simulink subsystem "WP07_PW"  (R2021b)
settings: Solver=VariableStepAuto  StartTime=0.0  StopTime=10.0  RelTol=1e-3
values from neighbouring files (symbols this model uses):
  Ctx_dcr_eol_dcr = [0.002858 0.002047 0.001273 0.000905] * 1.1    [Cal_WP07_Power.m]
  Ctx_dcr_eol_temp = [0 10 25 45]    [Cal_WP07_Power.m]
  Ctx_pow_chg_drt_coef = [0     0    0    1 1  0]    [Cal_WP07_Power.m]
  Ctx_pow_chg_drt_temp = [-22 -21.9  2.9  3 51 52]    [Cal_WP07_Power.m]
  Ctx_pow_dch_drt_coef = [0     0    0    1 1  0]    [Cal_WP07_Power.m]
  Ctx_pow_dch_drt_temp = [-22 -21.9  -0.1  0 51 52]    [Cal_WP07_Power.m]
  Ctx_pow_dch_soc_neg_pow_lim = [128 132 136 143 156]    [Cal_WP07_Power.m]
  Ctx_pow_dch_soc_neg_pow_now = [0.1 0.2 0.33 0.5 1]*183    [Cal_WP07_Power.m]
  Cxx_1cp_str = 183    [Cal_WP07_Power.m]
  Cxx_cell_t_fbdn_dch = -22    [Cal_WP07_Power.m]
  Cxx_cell_v_cut_off_chg = 4.1    [Cal_WP07_Power.m]
  Cxx_cell_v_cut_off_dch = 3.025    [Cal_WP07_Power.m]
  Cxx_cell_v_cut_off_dch_lowt = 3.2    [Cal_WP07_Power.m]
  Cxx_cell_v_fbdn_chg = 4.11    [Cal_WP07_Power.m]
  Cxx_cell_v_fbdn_dch = 3.015    [Cal_WP07_Power.m]
  Cxx_dcpm_r = 0.0464    [Cal_WP07_Power.m]
  Cxx_i_thrd_chg_act = 1    [Cal_WP07_Power.m]
  Cxx_i_thrd_dch_act = -1    [Cal_WP07_Power.m]
  Cxx_low_dch_hyst_off = 0    [Cal_WP07_Power.m]
  Cxx_low_dch_hyst_on = 3    [Cal_WP07_Power.m]
  Cxx_low_dch_pow = 5.5    [Cal_WP07_Power.m]
  Cxx_pow_dir_cf_time = 0.1    [Cal_WP07_Power.m]
  Cxx_pow_dir_chg = 2    [Cal_WP07_Power.m]
  Cxx_pow_dir_dch = 3    [Cal_WP07_Power.m]
  Cxx_pow_dir_init = 0    [Cal_WP07_Power.m]
  Cxx_pow_dir_stb = 1    [Cal_WP07_Power.m]
  Cxx_sch_pw = 0.1    [Cal_WP07_Power.m]
  Cxx_str_i_abs_max = 168    [Cal_WP07_Power.m]
undefined symbols (not defined in the file or in its folder): Cxx_cell_per_str, Nxx_m_1, Nxx_w_2_kw
libraries: Lib_MBD_Ext x4, simulink_extras x2
settings Model: Creator=DoHieuTrinh  LastModifiedBy=DoHieuTrinh

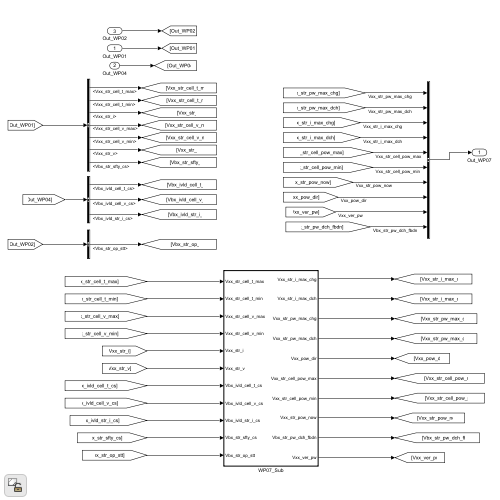
[thumbnail: Simulink's stored preview of the top-level diagram]
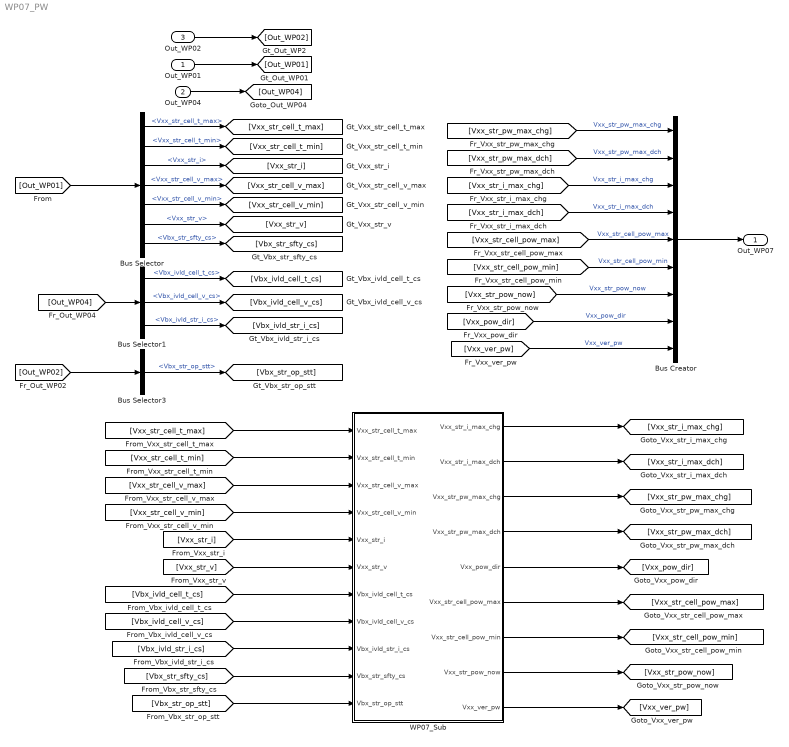
== system WP07_PW ==
  Out_WP01 : Inport
  Out_WP04 : Inport  Port=2
  Out_WP02 : Inport  Port=3
  Bus Creator : BusCreator  Inputs=9
  Bus Selector : BusSelector  OutputSignals=Vxx_str_cell_t_max,Vxx_str_cell_t_min,Vxx_str_i,Vxx_str_cell_v_max,Vxx_str_cell_v_min,Vxx_str_v,Vbx_str_sfty_cs
  Bus Selector1 : BusSelector  OutputSignals=Vbx_ivld_cell_t_cs,Vbx_ivld_cell_v_cs,Vbx_ivld_str_i_cs
  Bus Selector3 : BusSelector  OutputSignals=Vbx_str_op_stt
  WP07_Sub : Subsystem  TreatAsAtomicUnit=on  SystemSampleTime=0.1
  Out_WP07 : Outport
  wires:
  Bus Creator/1 -> Out_WP07/1
  [Vxx_str_pw_max_dch] -> Bus Creator/2  "Vxx_str_pw_max_dch"
  [Vxx_str_pw_max_chg] -> Bus Creator/1  "Vxx_str_pw_max_chg"
  [Out_WP01] -> Bus Selector/1
  Out_WP01/1 -> [Out_WP01]
  [Vxx_str_i_max_chg] -> Bus Creator/3  "Vxx_str_i_max_chg"
  [Vxx_str_i_max_dch] -> Bus Creator/4  "Vxx_str_i_max_dch"
  [Vxx_pow_dir] -> Bus Creator/8  "Vxx_pow_dir"
  WP07_Sub/1(Vxx_str_i_max_chg) -> [Vxx_str_i_max_chg]
  WP07_Sub/2(Vxx_str_i_max_dch) -> [Vxx_str_i_max_dch]
  WP07_Sub/3(Vxx_str_pw_max_chg) -> [Vxx_str_pw_max_chg]
  WP07_Sub/4(Vxx_str_pw_max_dch) -> [Vxx_str_pw_max_dch]
  WP07_Sub/5(Vxx_pow_dir) -> [Vxx_pow_dir]
  WP07_Sub/6(Vxx_str_cell_pow_max) -> [Vxx_str_cell_pow_max]
  WP07_Sub/7(Vxx_str_cell_pow_min) -> [Vxx_str_cell_pow_min]
  WP07_Sub/8(Vxx_str_pow_now) -> [Vxx_str_pow_now]
  [Vxx_str_cell_pow_max] -> Bus Creator/5  "Vxx_str_cell_pow_max"
  [Vxx_str_cell_pow_min] -> Bus Creator/6  "Vxx_str_cell_pow_min"
  [Vxx_str_pow_now] -> Bus Creator/7  "Vxx_str_pow_now"
  WP07_Sub/9(Vxx_ver_pw) -> [Vxx_ver_pw]
  [Vxx_ver_pw] -> Bus Creator/9  "Vxx_ver_pw"
  Out_WP04/1 -> [Out_WP04]
  [Out_WP04] -> Bus Selector1/1
  [Vxx_str_cell_t_max] -> WP07_Sub/1(Vxx_str_cell_t_max)
  [Vxx_str_cell_t_min] -> WP07_Sub/2(Vxx_str_cell_t_min)
  [Vxx_str_cell_v_max] -> WP07_Sub/3(Vxx_str_cell_v_max)
  [Vxx_str_cell_v_min] -> WP07_Sub/4(Vxx_str_cell_v_min)
  [Vxx_str_i] -> WP07_Sub/5(Vxx_str_i)
  [Vxx_str_v] -> WP07_Sub/6(Vxx_str_v)
  [Vbx_ivld_cell_t_cs] -> WP07_Sub/7(Vbx_ivld_cell_t_cs)
  [Vbx_ivld_cell_v_cs] -> WP07_Sub/8(Vbx_ivld_cell_v_cs)
  [Vbx_ivld_str_i_cs] -> WP07_Sub/9(Vbx_ivld_str_i_cs)
  Bus Selector/1 -> [Vxx_str_cell_t_max]  "<Vxx_str_cell_t_max>"
  Bus Selector/2 -> [Vxx_str_cell_t_min]  "<Vxx_str_cell_t_min>"
  Bus Selector/3 -> [Vxx_str_i]  "<Vxx_str_i>"
  Bus Selector/4 -> [Vxx_str_cell_v_max]  "<Vxx_str_cell_v_max>"
  Bus Selector/5 -> [Vxx_str_cell_v_min]  "<Vxx_str_cell_v_min>"
  Bus Selector/6 -> [Vxx_str_v]  "<Vxx_str_v>"
  Bus Selector1/1 -> [Vbx_ivld_cell_t_cs]  "<Vbx_ivld_cell_t_cs>"
  Bus Selector1/2 -> [Vbx_ivld_cell_v_cs]  "<Vbx_ivld_cell_v_cs>"
  Bus Selector1/3 -> [Vbx_ivld_str_i_cs]  "<Vbx_ivld_str_i_cs>"
  Bus Selector/7 -> [Vbx_str_sfty_cs]  "<Vbx_str_sfty_cs>"
  [Vbx_str_sfty_cs] -> WP07_Sub/10(Vbx_str_sfty_cs)
  [Vbx_str_op_stt] -> WP07_Sub/11(Vbx_str_op_stt)
  Bus Selector3/1 -> [Vbx_str_op_stt]  "<Vbx_str_op_stt>"
  [Out_WP02] -> Bus Selector3/1
  Out_WP02/1 -> [Out_WP02]

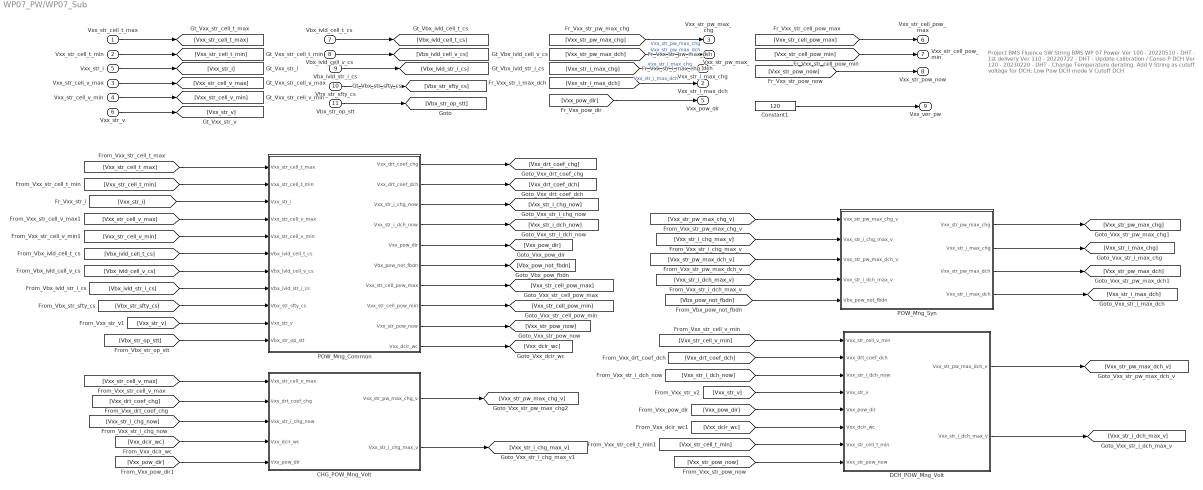
== system WP07_PW/WP07_Sub ==
  note: Project BMS Fluence
      | SW String BMS
      | WP 07 Power
      | Ver 100 - 20220510 - DHT - 1st delivery
      | Ver 110 - 20220722 - DHT - Update calibration / Conso P DCH
      | Ver 120 - 20230220 - DHT - Change Temperature derating.
      | Add V String as cutoff voltage for DCH; Low Pow DCH mode
      | V Cutoff DCH
  Vxx_str_cell_t_max : Inport
  Vxx_str_cell_t_min : Inport  Port=2
  Vxx_str_cell_v_max : Inport  Port=3
  Vxx_str_cell_v_min : Inport  Port=4
  Vxx_str_i : Inport  Port=5
  Vxx_str_v : Inport  Port=6
  Vbx_ivld_cell_t_cs : Inport  Port=7
  Vbx_ivld_cell_v_cs : Inport  Port=8
  Vbx_ivld_str_i_cs : Inport  Port=9
  Vbx_str_sfty_cs : Inport  Port=10
  Vbx_str_op_stt : Inport  Port=11
  CHG_POW_Mng_Volt : Subsystem
  Constant1 : Constant  Value=120  OutDataTypeStr=uint16
  DCH_POW_Mng_Volt : Subsystem
  POW_Mng_Common : Subsystem
  POW_Mng_Syn : Subsystem
  Vxx_str_i_max_chg : Outport
  Vxx_str_i_max_dch : Outport  Port=2
  Vxx_str_pw_max_chg : Outport  Port=3
  Vxx_str_pw_max_dch : Outport  Port=4
  Vxx_pow_dir : Outport  Port=5
  Vxx_str_cell_pow_max : Outport  Port=6
  Vxx_str_cell_pow_min : Outport  Port=7
  Vxx_str_pow_now : Outport  Port=8
  Vxx_ver_pw : Outport  Port=9
  wires:
  [Vxx_str_pow_now] -> DCH_POW_Mng_Volt/8(Vxx_str_pow_now)
  [Vxx_str_cell_t_min] -> DCH_POW_Mng_Volt/7(Vxx_str_cell_t_min)
  [Vxx_pow_dir] -> CHG_POW_Mng_Volt/5(Vxx_pow_dir)
  [Vxx_dcir_wc] -> DCH_POW_Mng_Volt/6(Vxx_dcir_wc)
  [Vxx_dcir_wc] -> CHG_POW_Mng_Volt/4(Vxx_dcir_wc)
  POW_Mng_Common/10(Vxx_dcir_wc) -> [Vxx_dcir_wc]
  [Vxx_pow_dir] -> DCH_POW_Mng_Volt/5(Vxx_pow_dir)
  [Vbx_str_op_stt] -> POW_Mng_Common/11(Vbx_str_op_stt)
  Vbx_str_op_stt/1 -> [Vbx_str_op_stt]
  [Vxx_str_v] -> POW_Mng_Common/10(Vxx_str_v)
  CHG_POW_Mng_Volt/2(Vxx_str_i_chg_max_v) -> [Vxx_str_i_chg_max_v]
  CHG_POW_Mng_Volt/1(Vxx_str_pw_max_chg_v) -> [Vxx_str_pw_max_chg_v]
  Vbx_str_sfty_cs/1 -> [Vbx_str_sfty_cs]
  [Vbx_str_sfty_cs] -> POW_Mng_Common/9(Vbx_str_sfty_cs)
  Vbx_ivld_str_i_cs/1 -> [Vbx_ivld_str_i_cs]
  Vbx_ivld_cell_v_cs/1 -> [Vbx_ivld_cell_v_cs]
  Vbx_ivld_cell_t_cs/1 -> [Vbx_ivld_cell_t_cs]
  [Vbx_ivld_str_i_cs] -> POW_Mng_Common/8(Vbx_ivld_str_i_cs)
  [Vbx_ivld_cell_v_cs] -> POW_Mng_Common/7(Vbx_ivld_cell_v_cs)
  [Vbx_ivld_cell_t_cs] -> POW_Mng_Common/6(Vbx_ivld_cell_t_cs)
  [Vxx_str_cell_v_min] -> POW_Mng_Common/5(Vxx_str_cell_v_min)
  [Vxx_str_cell_v_max] -> POW_Mng_Common/4(Vxx_str_cell_v_max)
  [Vxx_str_i] -> POW_Mng_Common/3(Vxx_str_i)
  [Vxx_str_cell_t_min] -> POW_Mng_Common/2(Vxx_str_cell_t_min)
  [Vxx_str_cell_t_max] -> POW_Mng_Common/1(Vxx_str_cell_t_max)
  Constant1/1 -> Vxx_ver_pw/1
  [Vxx_str_pow_now] -> Vxx_str_pow_now/1
  [Vxx_str_v] -> DCH_POW_Mng_Volt/4(Vxx_str_v)
  [Vxx_str_cell_pow_min] -> Vxx_str_cell_pow_min/1
  [Vxx_str_cell_pow_max] -> Vxx_str_cell_pow_max/1
  POW_Mng_Common/9(Vxx_str_pow_now) -> [Vxx_str_pow_now]
  POW_Mng_Common/8(Vxx_str_cell_pow_min) -> [Vxx_str_cell_pow_min]
  POW_Mng_Common/7(Vxx_str_cell_pow_max) -> [Vxx_str_cell_pow_max]
  [Vbx_pow_not_fbdn] -> POW_Mng_Syn/5(Vbx_pow_not_fbdn)
  POW_Mng_Common/6(Vbx_pow_not_fbdn) -> [Vbx_pow_not_fbdn]
  Vxx_str_v/1 -> [Vxx_str_v]
  [Vxx_pow_dir] -> Vxx_pow_dir/1
  POW_Mng_Common/5(Vxx_pow_dir) -> [Vxx_pow_dir]
  [Vxx_str_pw_max_dch] -> Vxx_str_pw_max_dch/1  "Vxx_str_pw_max_dch"
  [Vxx_str_pw_max_chg] -> Vxx_str_pw_max_chg/1  "Vxx_str_pw_max_chg"
  [Vxx_str_i_max_dch] -> Vxx_str_i_max_dch/1  "Vxx_str_i_max_dch"
  [Vxx_str_i_max_chg] -> Vxx_str_i_max_chg/1  "Vxx_str_i_max_chg"
  Vxx_str_i/1 -> [Vxx_str_i]
  Vxx_str_cell_v_min/1 -> [Vxx_str_cell_v_min]
  Vxx_str_cell_v_max/1 -> [Vxx_str_cell_v_max]
  Vxx_str_cell_t_min/1 -> [Vxx_str_cell_t_min]
  Vxx_str_cell_t_max/1 -> [Vxx_str_cell_t_max]
  [Vxx_drt_coef_dch] -> DCH_POW_Mng_Volt/2(Vxx_drt_coef_dch)
  POW_Mng_Syn/1(Vxx_str_pw_max_chg) -> [Vxx_str_pw_max_chg]
  POW_Mng_Syn/3(Vxx_str_pw_max_dch) -> [Vxx_str_pw_max_dch]
  POW_Mng_Common/3(Vxx_str_i_chg_now) -> [Vxx_str_i_chg_now]
  [Vxx_str_pw_max_dch_v] -> POW_Mng_Syn/3(Vxx_str_pw_max_dch_v)
  POW_Mng_Syn/2(Vxx_str_i_max_chg) -> [Vxx_str_i_max_chg]
  [Vxx_str_i_dch_max_v] -> POW_Mng_Syn/4(Vxx_str_i_dch_max_v)
  [Vxx_drt_coef_chg] -> CHG_POW_Mng_Volt/2(Vxx_drt_coef_chg)
  POW_Mng_Common/4(Vxx_str_i_dch_now) -> [Vxx_str_i_dch_now]
  [Vxx_str_pw_max_chg_v] -> POW_Mng_Syn/1(Vxx_str_pw_max_chg_v)
  [Vxx_str_i_chg_now] -> CHG_POW_Mng_Volt/3(Vxx_str_i_chg_now)
  [Vxx_str_i_dch_now] -> DCH_POW_Mng_Volt/3(Vxx_str_i_dch_now)
  POW_Mng_Syn/4(Vxx_str_i_max_dch) -> [Vxx_str_i_max_dch]
  [Vxx_str_i_chg_max_v] -> POW_Mng_Syn/2(Vxx_str_i_chg_max_v)
  POW_Mng_Common/1(Vxx_drt_coef_chg) -> [Vxx_drt_coef_chg]
  POW_Mng_Common/2(Vxx_drt_coef_dch) -> [Vxx_drt_coef_dch]
  DCH_POW_Mng_Volt/1(Vxx_str_pw_max_dch_v) -> [Vxx_str_pw_max_dch_v]
  DCH_POW_Mng_Volt/2(Vxx_str_i_dch_max_v) -> [Vxx_str_i_dch_max_v]
  [Vxx_str_cell_v_min] -> DCH_POW_Mng_Volt/1(Vxx_str_cell_v_min)
  [Vxx_str_cell_v_max] -> CHG_POW_Mng_Volt/1(Vxx_str_cell_v_max)

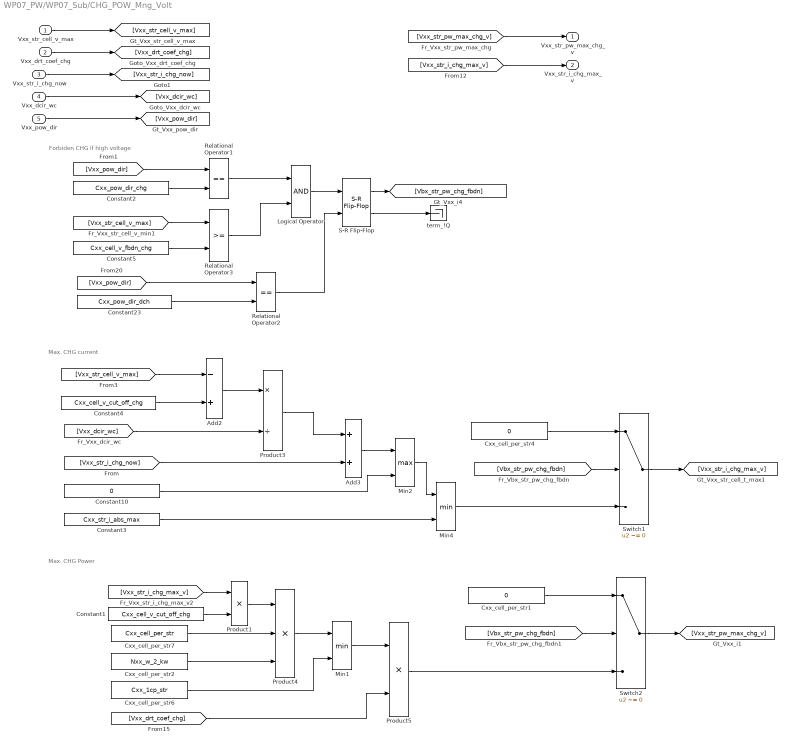
== system WP07_PW/WP07_Sub/CHG_POW_Mng_Volt ==
  note: Max. CHG current
  note: Max. CHG Power
  note: Forbiden CHG if high voltage
  Vxx_str_cell_v_max : Inport
  Vxx_drt_coef_chg : Inport  Port=2
  Vxx_str_i_chg_now : Inport  Port=3
  Vxx_dcir_wc : Inport  Port=4
  Vxx_pow_dir : Inport  Port=5
  Add2 : Sum  Inputs=-+
  Add3 : Sum
  Constant1 : Constant  Value=Cxx_cell_v_cut_off_chg  OutDataTypeStr=Inherit: Inherit via back propagation
  Constant10 : Constant  Value=0  OutDataTypeStr=Inherit: Inherit via back propagation
  Constant2 : Constant  Value=Cxx_pow_dir_chg  OutDataTypeStr=Inherit: Inherit via back propagation
  Constant23 : Constant  Value=Cxx_pow_dir_dch  OutDataTypeStr=Inherit: Inherit via back propagation
  Constant3 : Constant  Value=Cxx_str_i_abs_max  OutDataTypeStr=Inherit: Inherit via back propagation
  Constant4 : Constant  Value=Cxx_cell_v_cut_off_chg  OutDataTypeStr=Inherit: Inherit via back propagation
  Constant5 : Constant  Value=Cxx_cell_v_fbdn_chg  OutDataTypeStr=Inherit: Inherit via back propagation
  Cxx_cell_per_str1 : Constant  Value=0
  Cxx_cell_per_str2 : Constant  Value=Nxx_w_2_kw
  Cxx_cell_per_str4 : Constant  Value=0
  Cxx_cell_per_str6 : Constant  Value=Cxx_1cp_str
  Cxx_cell_per_str7 : Constant  Value=Cxx_cell_per_str
  Logical Operator : Logic  AllPortsSameDT=off  OutDataTypeStr=boolean
  Min1 : MinMax  Inputs=2
  Min2 : MinMax  Function=max  Inputs=2
  Min4 : MinMax  Inputs=2
  Product1 : Product
  Product3 : Product  Inputs=*/
  Product4 : Product  Inputs=3
  Product5 : Product
  Relational Operator1 : RelationalOperator  Operator===  OutDataTypeStr=boolean  RndMeth=Simplest
  Relational Operator2 : RelationalOperator  Operator===  OutDataTypeStr=boolean  RndMeth=Simplest
  Relational Operator3 : RelationalOperator  OutDataTypeStr=boolean  RndMeth=Simplest
  S-R Flip-Flop : simulink_extras/Flip Flops/S-R Flip-Flop  initial_condition=0
  Switch1 : Switch  Criteria=u2 ~= 0
  Switch2 : Switch  Criteria=u2 ~= 0
  term_!Q : Terminator
  Vxx_str_pw_max_chg_v : Outport
  Vxx_str_i_chg_max_v : Outport  Port=2
  wires:
  Relational Operator3/1 -> Logical Operator/2
  Product5/1 -> Switch2/3
  Switch2/1 -> [Vxx_str_pw_max_chg_v]
  Switch1/1 -> [Vxx_str_i_chg_max_v]
  [Vbx_str_pw_chg_fbdn] -> Switch2/2
  Cxx_cell_per_str1/1 -> Switch2/1
  Cxx_cell_per_str4/1 -> Switch1/1
  [Vbx_str_pw_chg_fbdn] -> Switch1/2
  Vxx_pow_dir/1 -> [Vxx_pow_dir]
  [Vxx_pow_dir] -> Relational Operator2/1
  [Vxx_str_cell_v_max] -> Relational Operator3/1
  Constant23/1 -> Relational Operator2/2
  Relational Operator2/1 -> S-R Flip-Flop/2
  Constant2/1 -> Relational Operator1/2
  S-R Flip-Flop/1 -> [Vbx_str_pw_chg_fbdn]
  S-R Flip-Flop/2 -> term_!Q/1
  [Vxx_pow_dir] -> Relational Operator1/1
  Logical Operator/1 -> S-R Flip-Flop/1
  Relational Operator1/1 -> Logical Operator/1
  Constant5/1 -> Relational Operator3/2
  Vxx_dcir_wc/1 -> [Vxx_dcir_wc]
  [Vxx_str_cell_v_max] -> Add2/1
  [Vxx_drt_coef_chg] -> Product5/2
  Min1/1 -> Product5/1
  Product4/1 -> Min1/1
  Cxx_cell_per_str2/1 -> Product4/3
  Cxx_cell_per_str7/1 -> Product4/2
  Product1/1 -> Product4/1
  Constant1/1 -> Product1/2
  [Vxx_str_i_chg_max_v] -> Product1/1
  Cxx_cell_per_str6/1 -> Min1/2
  Constant3/1 -> Min4/2
  Vxx_str_i_chg_now/1 -> [Vxx_str_i_chg_now]
  [Vxx_str_i_chg_max_v] -> Vxx_str_i_chg_max_v/1
  Vxx_drt_coef_chg/1 -> [Vxx_drt_coef_chg]
  Product3/1 -> Add3/1
  Vxx_str_cell_v_max/1 -> [Vxx_str_cell_v_max]
  Constant4/1 -> Add2/2
  [Vxx_dcir_wc] -> Product3/2
  Add2/1 -> Product3/1
  [Vxx_str_i_chg_now] -> Add3/2
  Add3/1 -> Min2/1
  Constant10/1 -> Min2/2
  [Vxx_str_pw_max_chg_v] -> Vxx_str_pw_max_chg_v/1
  Min4/1 -> Switch1/3
  Min2/1 -> Min4/1

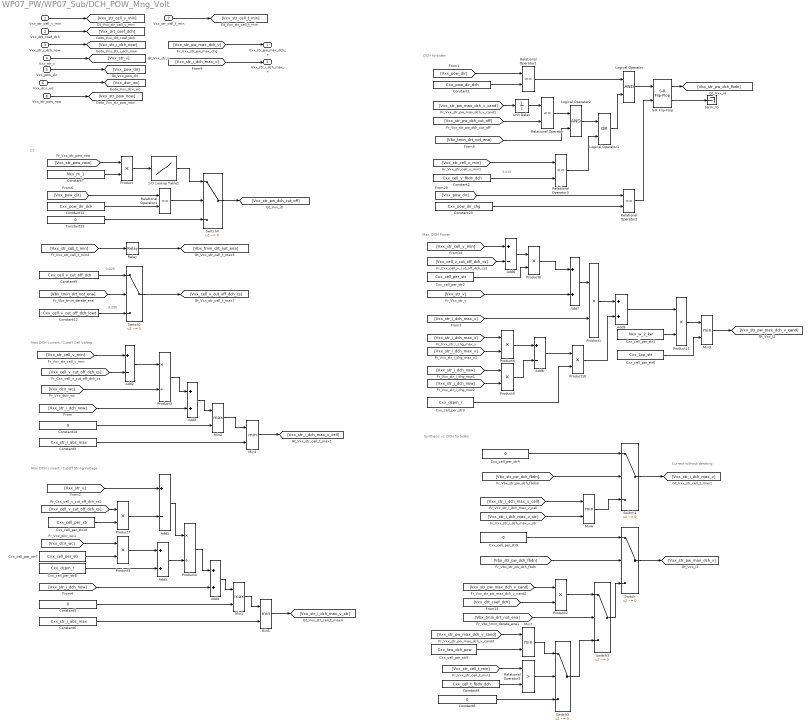
== system WP07_PW/WP07_Sub/DCH_POW_Mng_Volt ==
  note: Max DCH current / Cutoff String Voltage
  note: Max DCH current / Cutoff Cell Voltag
  note: Max. DCH Power
  note: DCH forbiden
  note: Synthesis vs. DCH forbiden
  note: CS
  note: Current without derating
  note: 3.015
  note: 3.025
  note: 3.200
  Vxx_str_cell_v_min : Inport
  Vxx_drt_coef_dch : Inport  Port=2
  Vxx_str_i_dch_now : Inport  Port=3
  Vxx_str_v : Inport  Port=4
  Vxx_pow_dir : Inport  Port=5
  Vxx_dcir_wc : Inport  Port=6
  Vxx_str_cell_t_min : Inport  Port=7
  Vxx_str_pow_now : Inport  Port=8
  1-D Lookup Table1 : Lookup_n-D  NumberOfTableDimensions=1  BreakpointsForDimension1=Ctx_pow_dch_soc_neg_pow_now  Table=Ctx_pow_dch_soc_neg_pow_lim  ExtrapMethod=Clip  UseLastTableValue=on  InternalRulePriority=Speed  RndMeth=Simplest  InputSameDT=on
  Add{1..2,6,8} (4 alike) : Sum  Inputs=+-
  Add{3..5,7,9} (5 alike) : Sum
  Constant1 : Constant  Value=Cxx_pow_dir_dch  OutDataTypeStr=Inherit: Inherit via back propagation
  Constant{5,8,10,13} (4 alike) : Constant  Value=0  OutDataTypeStr=Inherit: Inherit via back propagation
  Constant11 : Constant  Value=Cxx_pow_dir_dch  OutDataTypeStr=Inherit: Inherit via back propagation
  Constant12 : Constant  Value=Cxx_cell_v_cut_off_dch_lowt
  Constant2 : Constant  Value=Cxx_cell_v_fbdn_dch  OutDataTypeStr=Inherit: Inherit via back propagation
  Constant23 : Constant  Value=Cxx_pow_dir_chg  OutDataTypeStr=Inherit: Inherit via back propagation
  Constant3 : Constant  Value=Cxx_str_i_abs_max  OutDataTypeStr=Inherit: Inherit via back propagation
  Constant4 : Constant  Value=Cxx_cell_t_fbdn_dch  OutDataTypeStr=Inherit: Inherit via back propagation
  Constant6 : Constant  Value=Cxx_str_i_abs_max  OutDataTypeStr=Inherit: Inherit via back propagation
  Constant7 : Constant  Value=Nxx_m_1  OutDataTypeStr=Inherit: Inherit via back propagation
  Constant9 : Constant  Value=Cxx_cell_v_cut_off_dch
  Cxx_cell_per_str1 : Constant  Value=Nxx_w_2_kw
  Cxx_cell_per_str10 : Constant  Value=Cxx_cell_per_str
  Cxx_cell_per_str2 : Constant  Value=Cxx_cell_per_str
  Cxx_cell_per_str3 : Constant  Value=Cxx_dcpm_r
  Cxx_cell_per_str4 : Constant  Value=0
  Cxx_cell_per_str5 : Constant  Value=Cxx_low_dch_pow
  Cxx_cell_per_str6 : Constant  Value=Cxx_1cp_str
  Cxx_cell_per_str7 : Constant  Value=Cxx_cell_per_str
  Cxx_cell_per_str8 : Constant  Value=Cxx_dcpm_r
  Cxx_cell_per_str9 : Constant  Value=0
  Logical Operator : Logic  AllPortsSameDT=off  OutDataTypeStr=boolean
  Logical Operator1 : Logic  Operator=OR  AllPortsSameDT=off  OutDataTypeStr=boolean
  Logical Operator2 : Logic  AllPortsSameDT=off  OutDataTypeStr=boolean
  Min1 : MinMax  Function=max  Inputs=2
  Min2 : MinMax  Function=max  Inputs=2
  Min{3..7} (5 alike) : MinMax  Inputs=2
  Product{,1..2,5..11} (10 alike) : Product
  Product3 : Product  Inputs=*/
  Product4 : Product  Inputs=*/
  Relational Operator : RelationalOperator  Operator=<=  OutDataTypeStr=boolean  RndMeth=Simplest
  Relational Operator1 : RelationalOperator  Operator===  OutDataTypeStr=boolean  RndMeth=Simplest
  Relational Operator2 : RelationalOperator  Operator===  OutDataTypeStr=boolean  RndMeth=Simplest
  Relational Operator3 : RelationalOperator  Operator=<=  OutDataTypeStr=boolean  RndMeth=Simplest
  Relational Operator4 : RelationalOperator  Operator===  OutDataTypeStr=boolean  RndMeth=Simplest
  Relational Operator5 : RelationalOperator  Operator=>  OutDataTypeStr=boolean  RndMeth=Simplest
  Relay : Relay  OnSwitchValue=Cxx_low_dch_hyst_on  OffSwitchValue=Cxx_low_dch_hyst_off  OnOutputValue=true  OffOutputValue=false
  S-R Flip-Flop : simulink_extras/Flip Flops/S-R Flip-Flop  initial_condition=0
  Switch{,1..5} (6 alike) : Switch  Criteria=u2 ~= 0
  Unit Delay : UnitDelay  SampleTime=-1  HasFrameUpgradeWarning=on
  term_!Q : Terminator
  Vxx_str_pw_max_dch_v : Outport
  Vxx_str_i_dch_max_v : Outport  Port=2
  wires:
  Constant7/1 -> Product/2
  Product/1 -> 1-D Lookup Table1/1
  [Vxx_cell_v_cut_off_dch_cs] -> Add6/2
  Switch5/1 -> Switch3/3
  Constant8/1 -> Switch5/3
  Min7/1 -> Switch5/1
  Relational Operator5/1 -> Switch5/2
  [Vxx_str_cell_t_min] -> Relational Operator5/1
  Constant4/1 -> Relational Operator5/2
  [Vxx_str_pw_dch_cut_off] -> Relational Operator/2
  Switch4/1 -> [Vxx_str_pw_dch_cut_off]
  1-D Lookup Table1/1 -> Switch4/1
  [Vxx_str_pow_now] -> Product/1
  Constant13/1 -> Switch4/3
  Relational Operator4/1 -> Switch4/2
  Constant11/1 -> Relational Operator4/2
  [Vxx_pow_dir] -> Relational Operator4/1
  Vxx_str_pow_now/1 -> [Vxx_str_pow_now]
  Constant2/1 -> Relational Operator3/2
  [Vxx_cell_v_cut_off_dch_cs] -> Product7/1
  Cxx_cell_per_str10/1 -> Product7/2
  Logical Operator2/1 -> Logical Operator1/1
  [Vbx_tmin_drt_not_ena] -> Logical Operator2/2
  Relational Operator/1 -> Logical Operator2/1
  Switch3/1 -> Switch/3
  Cxx_cell_per_str5/1 -> Min7/2
  [Vxx_str_pw_max_dch_v_cand] -> Min7/1
  Product2/1 -> Switch3/1
  [Vxx_str_pw_max_dch_v_cand] -> Product2/1
  [Vbx_tmin_drt_not_ena] -> Switch3/2
  Min3/1 -> [Vxx_str_pw_max_dch_v_cand]
  [Vbx_tmin_drt_not_ena] -> Switch2/2
  Relay/1 -> [Vbx_tmin_drt_not_ena]
  [Vxx_cell_v_cut_off_dch_cs] -> Add2/2
  Vxx_str_cell_t_min/1 -> [Vxx_str_cell_t_min]
  Constant9/1 -> Switch2/1
  Switch2/1 -> [Vxx_cell_v_cut_off_dch_cs]
  Constant12/1 -> Switch2/3
  [Vxx_str_cell_t_min] -> Relay/1
  Min6/1 -> Switch1/3
  [Vxx_str_i_dch_max_v_cell] -> Min6/1
  [Vxx_str_i_dch_max_v_str] -> Min6/2
  Add5/1 -> Product4/2
  [Vxx_dcir_wc] -> Product5/1
  Product5/1 -> Add5/1
  Cxx_cell_per_str8/1 -> Add5/2
  Cxx_cell_per_str7/1 -> Product5/2
  Min1/1 -> Min5/1
  [Vxx_str_i_dch_now] -> Add4/2
  Constant5/1 -> Min1/2
  Constant6/1 -> Min5/2
  Min5/1 -> [Vxx_str_i_dch_max_v_str]
  Add4/1 -> Min1/1
  Product7/1 -> Add1/2
  Add1/1 -> Product4/1
  [Vxx_str_v] -> Add1/1
  Product4/1 -> Add4/1
  [Vxx_drt_coef_dch] -> Product2/2
  Unit Delay/1 -> Relational Operator/1
  [Vxx_str_pw_max_dch_v_cand] -> Unit Delay/1
  Switch1/1 -> [Vxx_str_i_dch_max_v]
  Cxx_cell_per_str4/1 -> Switch1/1
  [Vbx_str_pw_dch_fbdn] -> Switch1/2
  Logical Operator1/1 -> Logical Operator/2
  Relational Operator3/1 -> Logical Operator1/2
  [Vxx_str_cell_v_min] -> Relational Operator3/1
  Vxx_dcir_wc/1 -> [Vxx_dcir_wc]
  [Vbx_str_pw_dch_fbdn] -> Switch/2
  S-R Flip-Flop/1 -> [Vbx_str_pw_dch_fbdn]
  S-R Flip-Flop/2 -> term_!Q/1
  Logical Operator/1 -> S-R Flip-Flop/1
  Relational Operator1/1 -> Logical Operator/1
  [Vxx_pow_dir] -> Relational Operator1/1
  Constant1/1 -> Relational Operator1/2
  Vxx_pow_dir/1 -> [Vxx_pow_dir]
  Relational Operator2/1 -> S-R Flip-Flop/2
  Cxx_cell_per_str9/1 -> Switch/1
  Constant23/1 -> Relational Operator2/2
  [Vxx_pow_dir] -> Relational Operator2/1
  [Vxx_str_cell_v_min] -> Add2/1
  Switch/1 -> [Vxx_str_pw_max_dch_v]
  Product11/1 -> Min3/1
  Cxx_cell_per_str6/1 -> Min3/2
  Cxx_cell_per_str2/1 -> Product6/2
  Product6/1 -> Add7/1
  Add6/1 -> Product6/1
  Vxx_str_v/1 -> [Vxx_str_v]
  Cxx_cell_per_str3/1 -> Product10/2
  [Vxx_str_i_dch_now] -> Product9/1
  [Vxx_str_i_dch_max_v] -> Product1/2
  Product1/1 -> Add9/1
  [Vxx_str_i_dch_now] -> Product9/2
  Cxx_cell_per_str1/1 -> Product11/2
  Product8/1 -> Add8/1
  [Vxx_str_i_dch_max_v] -> Product8/1
  Add8/1 -> Product10/1
  [Vxx_str_v] -> Add7/2
  Product9/1 -> Add8/2
  [Vxx_str_i_dch_max_v] -> Product8/2
  Add7/1 -> Product1/1
  Add9/1 -> Product11/1
  Product10/1 -> Add9/2
  [Vxx_str_cell_v_min] -> Add6/1
  Constant3/1 -> Min4/2
  [Vxx_str_i_dch_max_v] -> Vxx_str_i_dch_max_v/1
  Vxx_str_i_dch_now/1 -> [Vxx_str_i_dch_now]
  Vxx_drt_coef_dch/1 -> [Vxx_drt_coef_dch]
  [Vxx_str_pw_max_dch_v] -> Vxx_str_pw_max_dch_v/1
  Constant10/1 -> Min2/2
  Add3/1 -> Min2/1
  [Vxx_str_i_dch_now] -> Add3/2
  Product3/1 -> Add3/1
  Add2/1 -> Product3/1
  [Vxx_dcir_wc] -> Product3/2
  Vxx_str_cell_v_min/1 -> [Vxx_str_cell_v_min]
  Min2/1 -> Min4/1
  Min4/1 -> [Vxx_str_i_dch_max_v_cell]

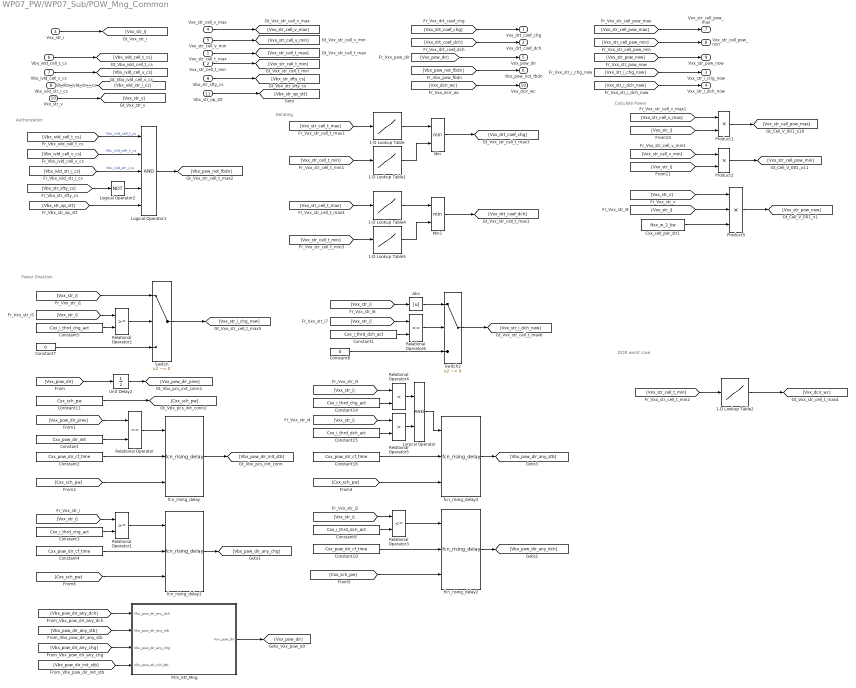
== system WP07_PW/WP07_Sub/POW_Mng_Common ==
  note: Calculate Power
  note: Derating
  note: Authorization
  note: Power Direction
  note: DCIR worst case
  Vxx_str_cell_t_max : Inport
  Vxx_str_cell_t_min : Inport  Port=2
  Vxx_str_i : Inport  Port=3
  Vxx_str_cell_v_max : Inport  Port=4
  Vxx_str_cell_v_min : Inport  Port=5
  Vbx_ivld_cell_t_cs : Inport  Port=6
  Vbx_ivld_cell_v_cs : Inport  Port=7
  Vbx_ivld_str_i_cs : Inport  Port=8
  Vbx_str_sfty_cs : Inport  Port=9
  Vxx_str_v : Inport  Port=10
  Vbx_str_op_stt : Inport  Port=11
  1-D Lookup Table : Lookup_n-D  NumberOfTableDimensions=1  BreakpointsForDimension1=Ctx_pow_chg_drt_temp  Table=Ctx_pow_chg_drt_coef  ExtrapMethod=Clip  UseLastTableValue=on  InternalRulePriority=Speed  RndMeth=Simplest  InputSameDT=on
  1-D Lookup Table1 : Lookup_n-D  NumberOfTableDimensions=1  BreakpointsForDimension1=Ctx_pow_chg_drt_temp  Table=Ctx_pow_chg_drt_coef  ExtrapMethod=Clip  UseLastTableValue=on  InternalRulePriority=Speed  RndMeth=Simplest  InputSameDT=on
  1-D Lookup Table2 : Lookup_n-D  NumberOfTableDimensions=1  BreakpointsForDimension1=Ctx_dcr_eol_temp  Table=Ctx_dcr_eol_dcr  ExtrapMethod=Clip  UseLastTableValue=on  InternalRulePriority=Speed  RndMeth=Simplest  InputSameDT=on
  1-D Lookup Table4 : Lookup_n-D  NumberOfTableDimensions=1  BreakpointsForDimension1=Ctx_pow_dch_drt_temp  Table=Ctx_pow_dch_drt_coef  ExtrapMethod=Clip  UseLastTableValue=on  InternalRulePriority=Speed  RndMeth=Simplest  InputSameDT=on
  1-D Lookup Table5 : Lookup_n-D  NumberOfTableDimensions=1  BreakpointsForDimension1=Ctx_pow_dch_drt_temp  Table=Ctx_pow_dch_drt_coef  ExtrapMethod=Clip  UseLastTableValue=on  InternalRulePriority=Speed  RndMeth=Simplest  InputSameDT=on
  Abs : Abs
  Constant : Constant  Value=Cxx_pow_dir_init
  Constant1 : Constant  Value=Cxx_i_thrd_dch_act
  Constant{2,4,10,16} (4 alike) : Constant  Value=Cxx_pow_dir_cf_time
  Constant11 : Constant  Value=Cxx_sch_pw
  Constant14 : Constant  Value=Cxx_i_thrd_chg_act
  Constant15 : Constant  Value=Cxx_i_thrd_dch_act
  Constant3 : Constant  Value=Cxx_i_thrd_chg_act
  Constant5 : Constant  Value=Cxx_i_thrd_chg_act
  Constant6 : Constant  Value=0
  Constant7 : Constant  Value=0
  Constant9 : Constant  Value=Cxx_i_thrd_dch_act
  Cxx_cell_per_str1 : Constant  Value=Nxx_w_2_kw
  Logical Operator : Logic  AllPortsSameDT=off  OutDataTypeStr=boolean
  Logical Operator1 : Logic  Inputs=5  AllPortsSameDT=off  OutDataTypeStr=boolean
  Logical Operator2 : Logic  Operator=NOT  AllPortsSameDT=off  OutDataTypeStr=boolean
  Min : MinMax  Inputs=2
  Min1 : MinMax  Inputs=2
  PCS_Stt_Mng : Stateflow chart  TreatAsAtomicUnit=on
  Product1 : Product
  Product2 : Product
  Product5 : Product  Inputs=3
  Relational Operator : RelationalOperator  Operator===  OutDataTypeStr=boolean  RndMeth=Simplest
  Relational Operator1 : RelationalOperator  OutDataTypeStr=boolean  RndMeth=Simplest
  Relational Operator2 : RelationalOperator  OutDataTypeStr=boolean  RndMeth=Simplest
  Relational Operator3 : RelationalOperator  Operator=<=  OutDataTypeStr=boolean  RndMeth=Simplest
  Relational Operator4 : RelationalOperator  Operator=<  OutDataTypeStr=boolean  RndMeth=Simplest
  Relational Operator5 : RelationalOperator  Operator=>  OutDataTypeStr=boolean  RndMeth=Simplest
  Relational Operator6 : RelationalOperator  Operator=<=  OutDataTypeStr=boolean  RndMeth=Simplest
  Switch : Switch  Criteria=u2 ~= 0
  Switch2 : Switch  Criteria=u2 ~= 0
  Unit Delay2 : UnitDelay  SampleTime=-1  HasFrameUpgradeWarning=on
  fcn_rising_delay{,1..3} (4 alike) : Lib_MBD_Ext/Timer/fcn_rising_delay  SystemSampleTime=-1  VariantActivationTime=update diagram  Latency=0  AutoFrameSizeCalculation=off
  Vxx_drt_coef_chg : Outport
  Vxx_drt_coef_dch : Outport  Port=2
  Vxx_str_i_chg_now : Outport  Port=3
  Vxx_str_i_dch_now : Outport  Port=4
  Vxx_pow_dir : Outport  Port=5
  Vbx_pow_not_fbdn : Outport  Port=6
  Vxx_str_cell_pow_max : Outport  Port=7
  Vxx_str_cell_pow_min : Outport  Port=8
  Vxx_str_pow_now : Outport  Port=9
  Vxx_dcir_wc : Outport  Port=10
  wires:
  Product5/1 -> [Vxx_str_pow_now]
  Cxx_cell_per_str1/1 -> Product5/3
  [Vxx_dcir_wc] -> Vxx_dcir_wc/1
  1-D Lookup Table2/1 -> [Vxx_dcir_wc]
  [Vxx_str_cell_t_min] -> 1-D Lookup Table2/1
  Constant1/1 -> Relational Operator6/2
  [Vxx_str_i] -> Relational Operator6/1
  Relational Operator2/1 -> Switch/2
  [Vxx_str_i] -> Relational Operator2/1
  Constant5/1 -> Relational Operator2/2
  [Vbx_str_op_stt] -> Logical Operator1/5
  Vbx_str_op_stt/1 -> [Vbx_str_op_stt]
  Constant11/1 -> [Cxx_sch_pw]
  Constant6/1 -> Switch2/3
  Abs/1 -> Switch2/1
  Vxx_str_v/1 -> [Vxx_str_v]
  [Vxx_str_v] -> Product5/1
  Logical Operator2/1 -> Logical Operator1/4
  [Vbx_str_sfty_cs] -> Logical Operator2/1
  Vbx_str_sfty_cs/1 -> [Vbx_str_sfty_cs]
  Vbx_ivld_str_i_cs/1 -> [Vbx_ivld_str_i_cs]
  Vbx_ivld_cell_v_cs/1 -> [Vbx_ivld_cell_v_cs]
  Vbx_ivld_cell_t_cs/1 -> [Vbx_ivld_cell_t_cs]
  [Vbx_ivld_str_i_cs] -> Logical Operator1/3  "Vbx_ivld_str_i_cs"
  [Vbx_ivld_cell_v_cs] -> Logical Operator1/2  "Vbx_ivld_cell_v_cs"
  [Vbx_ivld_cell_t_cs] -> Logical Operator1/1  "Vbx_ivld_cell_t_cs"
  [Vxx_str_i] -> Product5/2
  [Vxx_str_pow_now] -> Vxx_str_pow_now/1
  [Vxx_str_cell_pow_min] -> Vxx_str_cell_pow_min/1
  [Vxx_str_cell_pow_max] -> Vxx_str_cell_pow_max/1
  Vxx_str_cell_v_min/1 -> [Vxx_str_cell_v_min]
  Vxx_str_cell_v_max/1 -> [Vxx_str_cell_v_max]
  Product2/1 -> [Vxx_str_cell_pow_min]
  [Vxx_str_i] -> Product1/2
  [Vxx_str_cell_v_min] -> Product2/1
  [Vxx_str_i] -> Product2/2
  [Vxx_str_cell_v_max] -> Product1/1
  Product1/1 -> [Vxx_str_cell_pow_max]
  [Vbx_pow_not_fbdn] -> Vbx_pow_not_fbdn/1
  Logical Operator1/1 -> [Vbx_pow_not_fbdn]
  [Vxx_pow_dir] -> Vxx_pow_dir/1
  [Vxx_str_i_dch_now] -> Vxx_str_i_dch_now/1
  [Vxx_str_i_chg_now] -> Vxx_str_i_chg_now/1
  Relational Operator6/1 -> Switch2/2
  [Vxx_str_i] -> Abs/1
  Switch2/1 -> [Vxx_str_i_dch_now]
  Switch/1 -> [Vxx_str_i_chg_now]
  Constant7/1 -> Switch/3
  [Vxx_str_i] -> Switch/1
  [Vxx_drt_coef_dch] -> Vxx_drt_coef_dch/1
  1-D Lookup Table5/1 -> Min1/2
  [Vxx_str_cell_t_max] -> 1-D Lookup Table4/1
  1-D Lookup Table4/1 -> Min1/1
  Min1/1 -> [Vxx_drt_coef_dch]
  [Vxx_str_cell_t_min] -> 1-D Lookup Table5/1
  [Vxx_drt_coef_chg] -> Vxx_drt_coef_chg/1
  Logical Operator/1 -> fcn_rising_delay3/1
  fcn_rising_delay3/1 -> [Vbx_pow_dir_any_stb]
  [Cxx_sch_pw] -> fcn_rising_delay3/3
  Constant16/1 -> fcn_rising_delay3/2
  Relational Operator5/1 -> Logical Operator/2
  Relational Operator4/1 -> Logical Operator/1
  Constant15/1 -> Relational Operator5/2
  [Vxx_str_i] -> Relational Operator5/1
  [Vxx_str_i] -> Relational Operator4/1
  Constant14/1 -> Relational Operator4/2
  [Vxx_str_i] -> Relational Operator3/1
  Constant9/1 -> Relational Operator3/2
  Constant10/1 -> fcn_rising_delay2/2
  [Cxx_sch_pw] -> fcn_rising_delay2/3
  Relational Operator3/1 -> fcn_rising_delay2/1
  fcn_rising_delay2/1 -> [Vbx_pow_dir_any_dch]
  fcn_rising_delay1/1 -> [Vbx_pow_dir_any_chg]
  Relational Operator1/1 -> fcn_rising_delay1/1
  [Cxx_sch_pw] -> fcn_rising_delay1/3
  Constant4/1 -> fcn_rising_delay1/2
  Constant3/1 -> Relational Operator1/2
  [Vxx_pow_dir] -> Unit Delay2/1
  PCS_Stt_Mng/1(Vxx_pow_dir) -> [Vxx_pow_dir]
  [Vbx_pow_dir_init_stb] -> PCS_Stt_Mng/4(Vbx_pow_dir_init_stb)
  [Vbx_pow_dir_any_chg] -> PCS_Stt_Mng/3(Vbx_pow_dir_any_chg)
  [Vbx_pow_dir_any_stb] -> PCS_Stt_Mng/2(Vbx_pow_dir_any_stb)
  [Vbx_pow_dir_any_dch] -> PCS_Stt_Mng/1(Vbx_pow_dir_any_dch)
  Constant/1 -> Relational Operator/2
  fcn_rising_delay/1 -> [Vbx_pow_dir_init_stb]
  Relational Operator/1 -> fcn_rising_delay/1
  Constant2/1 -> fcn_rising_delay/2
  [Cxx_sch_pw] -> fcn_rising_delay/3
  [Vxx_pow_dir_prev] -> Relational Operator/1
  Unit Delay2/1 -> [Vxx_pow_dir_prev]
  Min/1 -> [Vxx_drt_coef_chg]
  1-D Lookup Table1/1 -> Min/2
  1-D Lookup Table/1 -> Min/1
  [Vxx_str_cell_t_min] -> 1-D Lookup Table1/1
  [Vxx_str_cell_t_max] -> 1-D Lookup Table/1
  [Vxx_str_i] -> Relational Operator1/1
  Vxx_str_i/1 -> [Vxx_str_i]
  Vxx_str_cell_t_min/1 -> [Vxx_str_cell_t_min]
  Vxx_str_cell_t_max/1 -> [Vxx_str_cell_t_max]

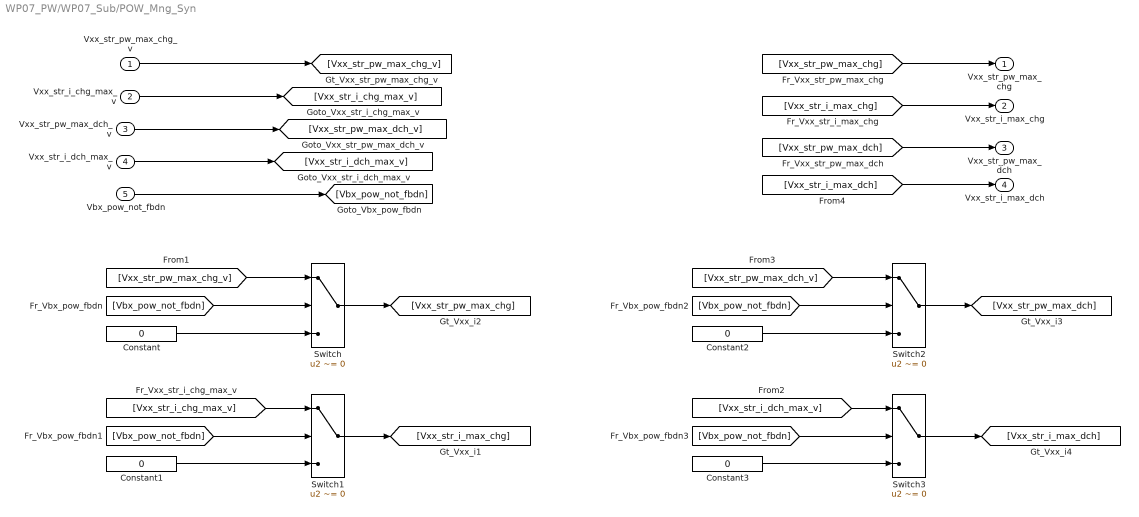
== system WP07_PW/WP07_Sub/POW_Mng_Syn ==
  Vxx_str_pw_max_chg_v : Inport
  Vxx_str_i_chg_max_v : Inport  Port=2
  Vxx_str_pw_max_dch_v : Inport  Port=3
  Vxx_str_i_dch_max_v : Inport  Port=4
  Vbx_pow_not_fbdn : Inport  Port=5
  Constant{,1..3} (4 alike) : Constant  Value=0
  Switch{,1..3} (4 alike) : Switch  Criteria=u2 ~= 0
  Vxx_str_pw_max_chg : Outport
  Vxx_str_i_max_chg : Outport  Port=2
  Vxx_str_pw_max_dch : Outport  Port=3
  Vxx_str_i_max_dch : Outport  Port=4
  wires:
  Switch3/1 -> [Vxx_str_i_max_dch]
  [Vxx_str_i_dch_max_v] -> Switch3/1
  Constant3/1 -> Switch3/3
  [Vbx_pow_not_fbdn] -> Switch3/2
  Switch2/1 -> [Vxx_str_pw_max_dch]
  [Vxx_str_pw_max_dch_v] -> Switch2/1
  [Vbx_pow_not_fbdn] -> Switch2/2
  Constant2/1 -> Switch2/3
  Switch1/1 -> [Vxx_str_i_max_chg]
  [Vxx_str_i_chg_max_v] -> Switch1/1
  [Vbx_pow_not_fbdn] -> Switch1/2
  Constant1/1 -> Switch1/3
  [Vxx_str_pw_max_chg_v] -> Switch/1
  Constant/1 -> Switch/3
  Switch/1 -> [Vxx_str_pw_max_chg]
  [Vbx_pow_not_fbdn] -> Switch/2
  Vbx_pow_not_fbdn/1 -> [Vbx_pow_not_fbdn]
  [Vxx_str_i_max_dch] -> Vxx_str_i_max_dch/1
  Vxx_str_i_dch_max_v/1 -> [Vxx_str_i_dch_max_v]
  Vxx_str_pw_max_dch_v/1 -> [Vxx_str_pw_max_dch_v]
  [Vxx_str_pw_max_dch] -> Vxx_str_pw_max_dch/1
  [Vxx_str_i_max_chg] -> Vxx_str_i_max_chg/1
  Vxx_str_i_chg_max_v/1 -> [Vxx_str_i_chg_max_v]
  Vxx_str_pw_max_chg_v/1 -> [Vxx_str_pw_max_chg_v]
  [Vxx_str_pw_max_chg] -> Vxx_str_pw_max_chg/1

== stateflow chart WP07_PW/WP07_Sub/POW_Mng_Common/PCS_Stt_Mng ==
  state Init
    entry:
    Vxx_pow_dir = Cxx_pow_dir_init;
  state Standby
    entry:
    Vxx_pow_dir = Cxx_pow_dir_stb;
  state Charge
    entry:
    Vxx_pow_dir = Cxx_pow_dir_chg;
  state Discharge
    entry:
    Vxx_pow_dir = Cxx_pow_dir_dch;
  (default) -> Init
  Init -> Standby : [Vbx_pow_dir_init_stb]
  Standby -> Charge [order 1] : [Vbx_pow_dir_any_chg]
  Standby -> Discharge [order 2] : [Vbx_pow_dir_any_dch]
  Charge -> Standby [order 1] : [Vbx_pow_dir_any_stb]
  Discharge -> Standby [order 1] : [Vbx_pow_dir_any_stb]
  Charge -> Discharge [order 2] : [Vbx_pow_dir_any_dch]
  Discharge -> Charge [order 2] : [Vbx_pow_dir_any_chg]
  data: Cxx_pow_dir_stb parameter; Cxx_pow_dir_init parameter; Cxx_pow_dir_chg parameter; Cxx_pow_dir_dch parameter; Vbx_pow_dir_any_dch input; Vbx_pow_dir_any_stb input; Vbx_pow_dir_any_chg input; Vbx_pow_dir_init_stb input; Vxx_pow_dir output
